simulink model "test_fk"  (R2022a)
settings: Solver=VariableStepAuto  StartTime=0.0  StopTime=10.0  RelTol=1e-3
libraries: simulink_extras x9
settings Model: Creator=Dell  LastModifiedBy=Dell

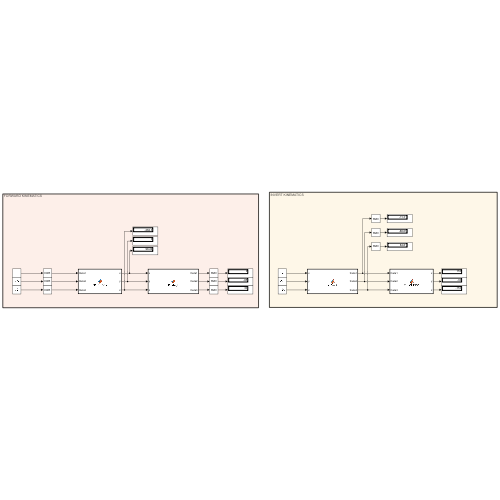
[thumbnail: Simulink's stored preview of the top-level diagram]
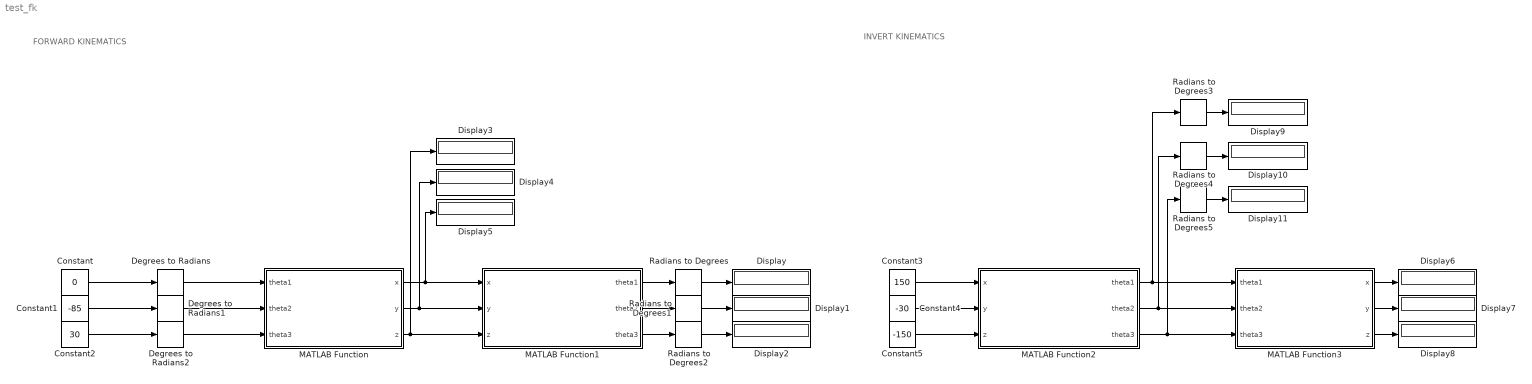
== system test_fk ==
  note: INVERT KINEMATICS
  note: FORWARD KINEMATICS
  Constant : Constant  Value=0
  Constant1 : Constant  Value=-85
  Constant2 : Constant  Value=30
  Constant3 : Constant  Value=150
  Constant4 : Constant  Value=-30
  Constant5 : Constant  Value=-150
  Degrees to Radians : simulink_extras/Transformations/Degrees to Radians
  Degrees to Radians1 : simulink_extras/Transformations/Degrees to Radians
  Degrees to Radians2 : simulink_extras/Transformations/Degrees to Radians
  Display{,1..11} (12 alike) : Display
  MATLAB Function : MATLAB Function  TreatAsAtomicUnit=on
  MATLAB Function1 : MATLAB Function  TreatAsAtomicUnit=on
  MATLAB Function2 : MATLAB Function  TreatAsAtomicUnit=on
  MATLAB Function3 : MATLAB Function  TreatAsAtomicUnit=on
  Radians to Degrees{,1..5} (6 alike) : simulink_extras/Transformations/Radians to Degrees
  wires:
  Constant/1 -> Degrees to Radians/1
  Constant1/1 -> Degrees to Radians1/1
  Constant2/1 -> Degrees to Radians2/1
  MATLAB Function/1(x) -> Display5/1, MATLAB Function1/1(x)
  MATLAB Function/2(y) -> Display4/1, MATLAB Function1/2(y)
  MATLAB Function1/1(theta1) -> Radians to Degrees/1
  MATLAB Function1/2(theta2) -> Radians to Degrees1/1
  MATLAB Function1/3(theta3) -> Radians to Degrees2/1
  MATLAB Function/3(z) -> Display3/1, MATLAB Function1/3(z)
  Degrees to Radians/1 -> MATLAB Function/1(theta1)
  Degrees to Radians1/1 -> MATLAB Function/2(theta2)
  Degrees to Radians2/1 -> MATLAB Function/3(theta3)
  Radians to Degrees/1 -> Display/1
  Radians to Degrees1/1 -> Display1/1
  Radians to Degrees2/1 -> Display2/1
  MATLAB Function2/1(theta1) -> MATLAB Function3/1(theta1), Radians to Degrees3/1
  MATLAB Function2/2(theta2) -> MATLAB Function3/2(theta2), Radians to Degrees4/1
  MATLAB Function2/3(theta3) -> MATLAB Function3/3(theta3), Radians to Degrees5/1
  Constant3/1 -> MATLAB Function2/1(x)
  Constant4/1 -> MATLAB Function2/2(y)
  Constant5/1 -> MATLAB Function2/3(z)
  MATLAB Function3/1(x) -> Display6/1
  MATLAB Function3/2(y) -> Display7/1
  MATLAB Function3/3(z) -> Display8/1
  Radians to Degrees3/1 -> Display9/1
  Radians to Degrees4/1 -> Display10/1
  Radians to Degrees5/1 -> Display11/1

== matlab function test_fk/MATLAB Function1 ==
  data: x input; theta1 output; y input; z input; theta2 output; theta3 output
function [theta1,theta2,theta3] = IK_Magic(x,y,z)
%% Programmed By Nguyen Trong Tin && Nguyen Tai Tue
l2 = 140;
l3 = 150;

theta1  = atan2(0,1)-atan2((-y/sqrt(x^2+y^2)),(x/sqrt(x^2+y^2)));

a = -2*z*l2;
b = -2*l2*(x*cos(theta1)+y*sin(theta1))
d = l3^2 - (x*cos(theta1)+y*sin(theta1))^2 -z^2 - l2^2;

theta2 = atan2((d/(sqrt(a^2+b^2))),-sqrt((a^2+b^2-d^2)/(a^2+b^2))) - atan2((b/sqrt(a^2+b^2)),(a/sqrt(a^2+b^2)))

s23 = (z-l2*sin(theta2))/l3;

c23 = sqrt(1-s23^2)

theta3 = atan2(s23,c23) - theta2


end

== matlab function test_fk/MATLAB Function ==
  data: x output; theta1 input; y output; theta2 input; theta3 input; z output
function [x,y,z] = FK_CHECK(theta1,theta2,theta3)
%% Programmed By Nguyen Trong Tin && Nguyen Tai Tue
l2 = 140;
l3 = 150;

x = l3*cos(theta1)*cos(theta2+theta3)+l2*cos(theta1)*cos(theta2)
y = l3*sin(theta1)*cos(theta2+theta3)+l2*sin(theta1)*cos(theta2)
z = l3*sin(theta2+theta3) + l2*sin(theta2)

end

== matlab function test_fk/MATLAB Function2 ==
  data: x input; theta1 output; y input; z input; theta2 output; theta3 output
function [theta1,theta2,theta3] = IK_Magic(x,y,z)

l2 = 140;
l3 = 150;

theta1  = atan2(0,1)-atan2((-y/sqrt(x^2+y^2)),(x/sqrt(x^2+y^2)));

a = -2*z*l2;
b = -2*l2*(x*cos(theta1)+y*sin(theta1))
d = l3^2 - (x*cos(theta1)+y*sin(theta1))^2 -z^2 - l2^2;

theta2 = atan2((d/(sqrt(a^2+b^2))),-sqrt((a^2+b^2-d^2)/(a^2+b^2))) - atan2((b/sqrt(a^2+b^2)),(a/sqrt(a^2+b^2)))

s23 = (z-l2*sin(theta2))/l3;

c23 = sqrt(1-s23^2)

theta3 = atan2(s23,c23) - theta2


end

== matlab function test_fk/MATLAB Function3 ==
  data: x output; theta1 input; y output; theta2 input; theta3 input; z output
function [x,y,z] = FK_CHECK(theta1,theta2,theta3)

l2 = 140;
l3 = 150;

x = l3*cos(theta1)*cos(theta2+theta3)+l2*cos(theta1)*cos(theta2)
y = l3*sin(theta1)*cos(theta2+theta3)+l2*sin(theta1)*cos(theta2)
z = l3*sin(theta2+theta3) + l2*sin(theta2)

end
